simulink model "Quadrotor_Control"  (R2024a)
settings: Solver=ode4  StartTime=0.0  StopTime=15  FixedStep=0.001  RelTol=1e-3
InitFcn:
  | fp=get_param(bdroot,'Filename');p=fileparts(fp);if ~isempty(p), addpath(p); end
settings Model: Creator=Lenovo  LastModifiedBy=Lenovo

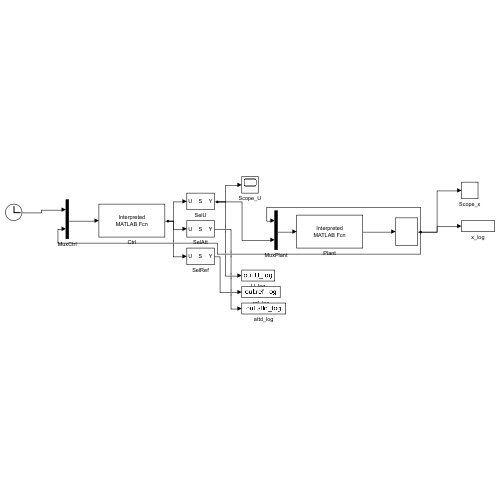
[thumbnail: Simulink's stored preview of the top-level diagram]
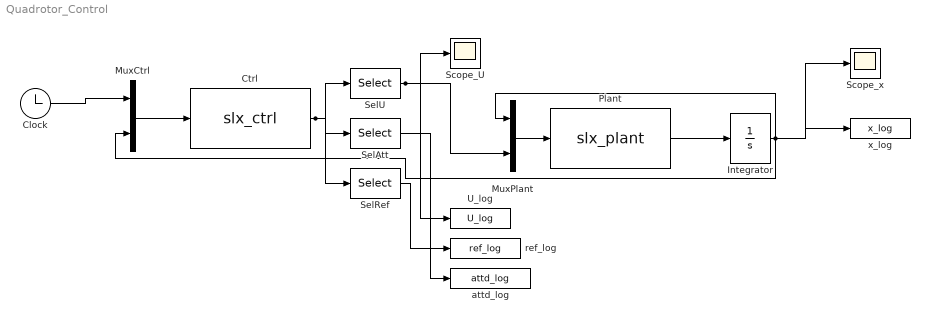
== system Quadrotor_Control ==
  Clock : Clock
  Ctrl : MATLABFcn  MATLABFcn=slx_ctrl  OutputDimensions=10
  Integrator : Integrator  InitialCondition=[0;0;0.05;0;0;0;0;0;0;0;0;0]
  MuxCtrl : Mux  Inputs=2
  MuxPlant : Mux  Inputs=2
  Plant : MATLABFcn  MATLABFcn=slx_plant  OutputDimensions=12
  Scope_U : Scope
  Scope_x : Scope
  SelAtt : Selector  InputPortWidth=10  IndexOptions=Index vector (dialog)  Indices=5:7  OutputSizes=1
  SelRef : Selector  InputPortWidth=10  IndexOptions=Index vector (dialog)  Indices=8:10  OutputSizes=1
  SelU : Selector  InputPortWidth=10  IndexOptions=Index vector (dialog)  Indices=1:4  OutputSizes=1
  U_log : ToWorkspace  VariableName=U_log  SaveFormat=Timeseries  SampleTime=-1
  attd_log : ToWorkspace  VariableName=attd_log  SaveFormat=Timeseries  SampleTime=-1
  ref_log : ToWorkspace  VariableName=ref_log  SaveFormat=Timeseries  SampleTime=-1
  x_log : ToWorkspace  VariableName=x_log  SaveFormat=Timeseries  SampleTime=-1
  wires:
  Clock/1 -> MuxCtrl/1
  Integrator/1 -> MuxCtrl/2, MuxPlant/1, Scope_x/1, x_log/1
  MuxCtrl/1 -> Ctrl/1
  Ctrl/1 -> SelU/1, SelAtt/1, SelRef/1
  SelU/1 -> MuxPlant/2, Scope_U/1, U_log/1
  MuxPlant/1 -> Plant/1
  Plant/1 -> Integrator/1
  SelRef/1 -> ref_log/1
  SelAtt/1 -> attd_log/1
